simulink model "QuinticTest"  (R2014a)
settings: Solver=ode8  StartTime=0.0  StopTime=43  FixedStep=1e-3  RelTol=1e-3
libraries: simulink x1
settings Model: Creator=Administrator  LastModifiedBy=Administrator

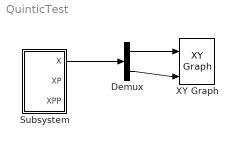
== system QuinticTest ==
  Demux : Demux  Outputs=2
  Subsystem : Subsystem
  XY Graph : simulink/Sinks/XY Graph  xmin=-1  xmax=1  ymin=-1  ymax=1  st=-1
  wires:
  Subsystem/1(X) -> Demux/1
  Demux/2 -> XY Graph/2
  Demux/1 -> XY Graph/1

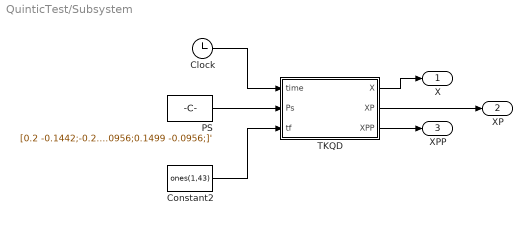
== system QuinticTest/Subsystem ==
  Clock : Clock
  Constant2 : Constant  Value=ones(1,43)
  PS : Constant  Value=[0.2 -0.1442;-0.2847 -0.0956;-0.2879 0.0916;-0.2673 0.0916;-0.2641 -0.0755;-0.1927 -0.0735;-0.1927 -0.0956;-0.2863 -0.0956;-0.1832 -0.0976;-0.1277 0.0936;-0.1087 0.0916;-0.0436 -0.0956;-0.0627 -0.0956;-0.0849 -0.0352;-0.1451 -0.0372;-0.1594 -0.0936;-0.1816 -0.0936;-0.0262 -0.0996;-0.0262 0.0936; 0.0040 0.0936; 0.0452 -0.0654; 0.0880 0.0916; 0.1134 0.0916; 0.1134 -0.0976; 0.0975 -0.0976; 0.0991 0.0574; 0.0531 -0.0956;0.0341 -0.0956;-0.0071 0.0614;-0.0087 -0.0956;-0.0262 -0.0956; 0.1499 -0.0956; 0.1499 0.0936; 0.2593 0.0936; 0.2578 0.0735; 0.1689 0.0735; 0.1689 0.0131; 0.2530 0.0131; 0.2530 -0.0070; 0.1705 -0.0070; 0.1721 -0.0775; 0.2625 -0.0775; 0.2625 -0.0956;0.1499 -0.0956;]'
  TKQD : MATLAB Function  TreatAsAtomicUnit=on
  X : Outport
  XP : Outport  Port=2
  XPP : Outport  Port=3
  wires:
  TKQD/2(XP) -> XP/1
  TKQD/3(XPP) -> XPP/1
  Clock/1 -> TKQD/1(time)
  TKQD/1(X) -> X/1
  PS/1 -> TKQD/2(Ps)
  Constant2/1 -> TKQD/3(tf)

== matlab function QuinticTest/Subsystem/TKQD ==
  data: time input; X output; Ps input; tf input; XP output; XPP output
function [X,XP,XPP] = Quintic(time,Ps,tf)
% Calculate trajectory using Quintic polynomial
% r=10*(t/tf)^3-15*(t/tf)^4+6*(t/tf)^5;
% time is clock input
% Ps is the list of point = [P1 P2...]
% tf is the finish time for each interval
n=length(tf);
[k,tk_1] = find(time,tf,n);
if(k==1)
    t=min(time/tf(1),1);
else
    t = min((time-tk_1)/tf(k),1);
end
r=10*t^3-15*t^4+6*t^5;
rd=30*t^2-60*t^3+30*t^4;
r2d=60*t-180*t^2+120*t^3;
D=Ps(:,k+1)-Ps(:,k);
X=Ps(:,k)+r*D;
XP=rd*D;
XPP=r2d*D;
function [k,tk_1]=find(time,tf,n)
t=0;
k=n;
for i=1:n
    tk=t+tf(i);
    if(t<=time)&&(time<tk)
        k=i;
        break;
    end
    t=tk;
    if(i==n)
        t=tk-tf(n);
    end
end
tk_1=t;
